simulink model "model_C5"  (R2019b)
settings: Solver=VariableStepAuto  StartTime=0.0  StopTime=3  RelTol=1e-3
libraries: simulink_extras x6
settings Model: Creator=vladg  LastModifiedBy=vladg

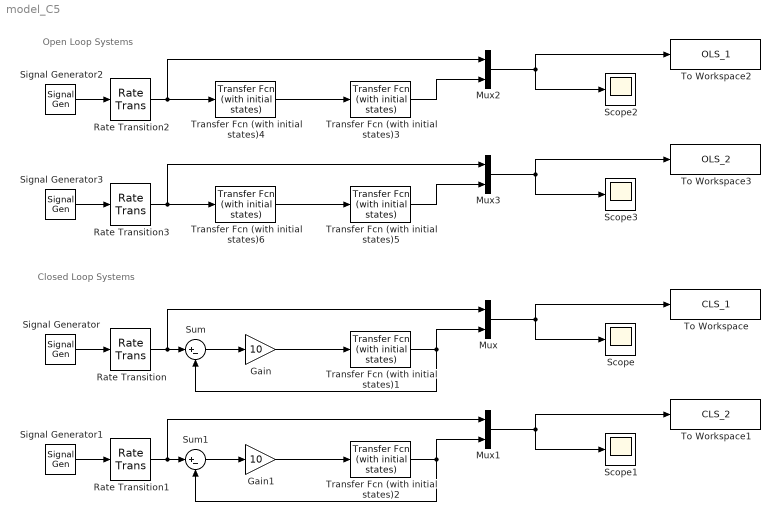
== system model_C5 ==
  note: Open Loop Systems
  note: Closed Loop Systems
  Gain : Gain  Gain=10
  Gain1 : Gain  Gain=10
  Mux{,1..3} (4 alike) : Mux  Inputs=2
  Rate Transition{,1..3} (4 alike) : RateTransition  OutPortSampleTime=0.001
  Scope{,1..3} (4 alike) : Scope
  Signal Generator{,1..3} (4 alike) : SignalGenerator  WaveForm=square  Frequency=0.5
  Sum : Sum  Inputs=|+-
  Sum1 : Sum  Inputs=|+-
  To Workspace : ToWorkspace  VariableName=CLS_1  SaveFormat=Timeseries  SampleTime=-1
  To Workspace1 : ToWorkspace  VariableName=CLS_2  SaveFormat=Timeseries  SampleTime=-1
  To Workspace2 : ToWorkspace  VariableName=OLS_1  SaveFormat=Timeseries  SampleTime=-1
  To Workspace3 : ToWorkspace  VariableName=OLS_2  SaveFormat=Timeseries  SampleTime=-1
  Transfer Fcn (with initial states)1 : simulink_extras/Additional Linear/Transfer Fcn (with initial states)  N=[1]  D="[1  0.5]"  X0=0
  Transfer Fcn (with initial states)2 : simulink_extras/Additional Linear/Transfer Fcn (with initial states)  N=[0.5]  D="[1  1]"  X0=0
  Transfer Fcn (with initial states)3 : simulink_extras/Additional Linear/Transfer Fcn (with initial states)  N=[1]  D="[1  1]"  X0=0
  Transfer Fcn (with initial states)4 : simulink_extras/Additional Linear/Transfer Fcn (with initial states)  N=[1 1]  D="[0.1  1]"  X0=0
  Transfer Fcn (with initial states)5 : simulink_extras/Additional Linear/Transfer Fcn (with initial states)  N=[1]  D="[1  1]"  X0=0
  Transfer Fcn (with initial states)6 : simulink_extras/Additional Linear/Transfer Fcn (with initial states)  N=[1 1]  D="[0.1  1]"  X0=0
  wires:
  Gain/1 -> Transfer Fcn (with initial states)1/1
  Transfer Fcn (with initial states)1/1 -> Sum/2, Mux/2
  Mux/1 -> Scope/1, To Workspace/1
  Signal Generator/1 -> Rate Transition/1
  Rate Transition/1 -> Mux/1, Sum/1
  Sum/1 -> Gain/1
  Sum1/1 -> Gain1/1
  Signal Generator1/1 -> Rate Transition1/1
  Rate Transition1/1 -> Mux1/1, Sum1/1
  Mux1/1 -> Scope1/1, To Workspace1/1
  Gain1/1 -> Transfer Fcn (with initial states)2/1
  Transfer Fcn (with initial states)2/1 -> Sum1/2, Mux1/2
  Signal Generator2/1 -> Rate Transition2/1
  Rate Transition2/1 -> Transfer Fcn (with initial states)4/1, Mux2/1
  Mux2/1 -> Scope2/1, To Workspace2/1
  Transfer Fcn (with initial states)4/1 -> Transfer Fcn (with initial states)3/1
  Transfer Fcn (with initial states)3/1 -> Mux2/2
  Transfer Fcn (with initial states)5/1 -> Mux3/2
  Rate Transition3/1 -> Transfer Fcn (with initial states)6/1, Mux3/1
  Signal Generator3/1 -> Rate Transition3/1
  Mux3/1 -> Scope3/1, To Workspace3/1
  Transfer Fcn (with initial states)6/1 -> Transfer Fcn (with initial states)5/1
